simulink library "LatchUtilities"  (R2021b)
settings: Solver=VariableStepAuto  StartTime=0.0  StopTime=10.0  RelTol=1e-3
settings Model: Creator=david  LastModifiedBy=david

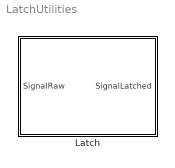
== system LatchUtilities ==
  Latch : Subsystem  mask{LatchTime=3}
      mask prompts: LatchTime "Latch time in seconds"

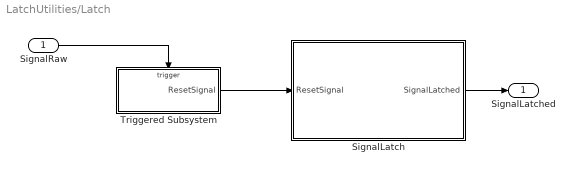
== system LatchUtilities/Latch ==
  SignalRaw : Inport  RequirementInfo={} %GIDa_c723fe9f_d72e_41d0_9824_e002adb82799  OutDataTypeStr=boolean
  SignalLatch : Stateflow chart  RequirementInfo={} %GIDa_48dfe4d5_e668_4584_aa00_8b63795508db  TreatAsAtomicUnit=on
  Triggered Subsystem : Subsystem  TreatAsAtomicUnit=on
  SignalLatched : Outport  RequirementInfo={} %GIDa_b045b639_6ae2_40e4_b241_c838abc0f670  OutDataTypeStr=boolean
  wires:
  SignalRaw/1 -> Triggered Subsystem/Trigger
  SignalLatch/1(SignalLatched) -> SignalLatched/1
  Triggered Subsystem/1(ResetSignal) -> SignalLatch/1(ResetSignal)

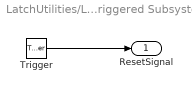
== system LatchUtilities/Latch/Triggered Subsystem ==
  Trigger : TriggerPort  TriggerType=either  VariantControl=(inherit)  ShowOutputPort=on  OutputDataType=int8
  ResetSignal : Outport
  wires:
  Trigger/1 -> ResetSignal/1

== stateflow chart LatchUtilities/Latch/SignalLatch ==
  state SignalResetState
    entry:
    ResetSignalCurrent = ResetSignal;
    SignalLatched = false;
  state SignalLatchedState
    entry:
    SignalLatched = true;
  (default) -> SignalResetState
  SignalResetState -> (junction 27) : [ResetSignal == ResetSignalCurrent]
  (junction 27) -> SignalResetState [order 2] : [ResetSignal ~= ResetSignalCurrent]
  SignalLatchedState -> SignalResetState : [ResetSignal ~= ResetSignalCurrent]
  (junction 27) -> SignalLatchedState [order 1] : [after(LatchTime, sec)]
  data: ResetSignalCurrent local; SignalLatched output; ResetSignal input; LatchTime parameter
